simulink model "pmsm_model_dq"  (R2023b)
settings: Solver=VariableStepAuto  StartTime=0.0  StopTime=10.0  RelTol=1e-3
values from neighbouring files (symbols this model uses):
  B = 0.0000028    (= 2.8e-06)    [pm_params.m]
  J = 0.00016    [pm_params.m]
  Ld = 0.0057    [pm_params.m]
  Lq = 0.0125    [pm_params.m]
  pole = 4    [pm_params.m]
  Rs = 1.2    [pm_params.m]
undefined symbols (not defined in the file or in its folder): Lambda_f
settings Model: Creator=Yang  LastModifiedBy=Yang

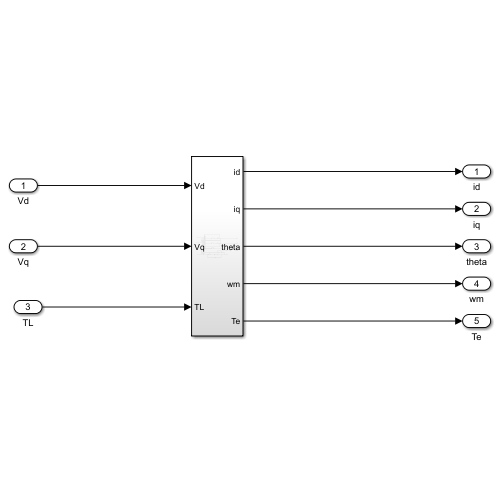
[thumbnail: Simulink's stored preview of the top-level diagram]
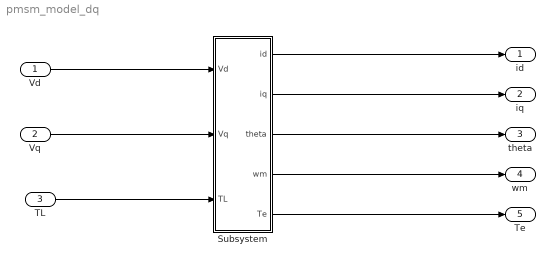
== system pmsm_model_dq ==
  Vd : Inport
  Vq : Inport  Port=2
  TL : Inport  Port=3
  Subsystem : Subsystem
  id : Outport
  iq : Outport  Port=2
  theta : Outport  Port=3
  wm : Outport  Port=4
  Te : Outport  Port=5
  wires:
  Vd/1 -> Subsystem/1(Vd)
  Vq/1 -> Subsystem/2(Vq)
  TL/1 -> Subsystem/3(TL)
  Subsystem/1(id) -> id/1
  Subsystem/2(iq) -> iq/1
  Subsystem/3(theta) -> theta/1
  Subsystem/4(wm) -> wm/1
  Subsystem/5(Te) -> Te/1

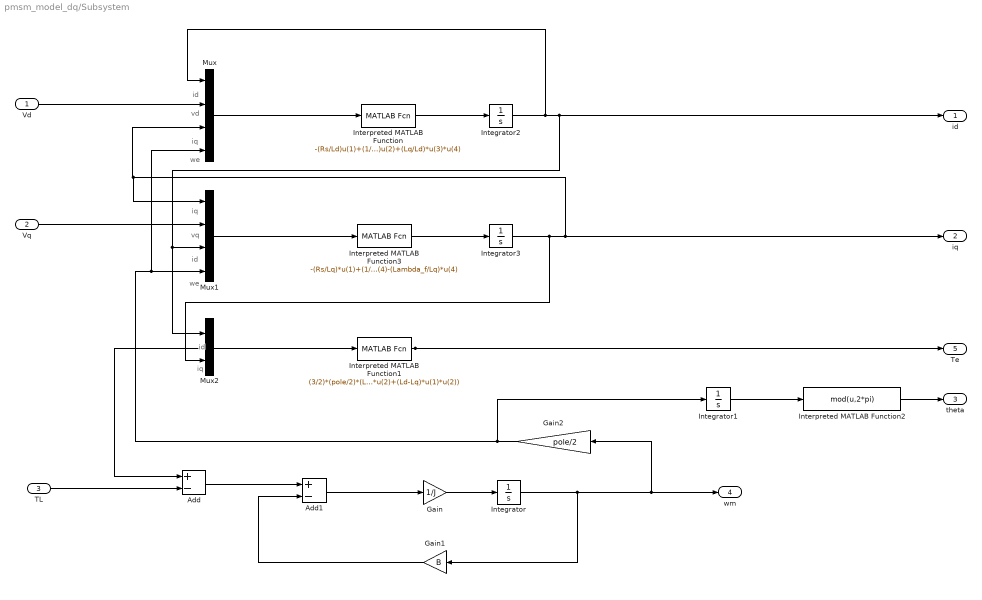
== system pmsm_model_dq/Subsystem ==
  note: iq
  note: id
  note: we
  note: id
  note: vq
  note: iq
  note: we
  note: iq
  note: vd
  note: id
  Vd : Inport
  Vq : Inport  Port=2
  TL : Inport  Port=3
  Add : Sum  Inputs=+-
  Add1 : Sum  Inputs=+-
  Gain : Gain  Gain=1/J
  Gain1 : Gain  Gain=B
  Gain2 : Gain  Gain=pole/2
  Integrator{,1..3} (4 alike) : Integrator
  Interpreted MATLAB Function : MATLABFcn  MATLABFcn=-(Rs/Ld)u(1)+(1/Ld)u(2)+(Lq/Ld)*u(3)*u(4)
  Interpreted MATLAB Function1 : MATLABFcn  MATLABFcn=(3/2)*(pole/2)*(Lambda_f*u(2)+(Ld-Lq)*u(1)*u(2))
  Interpreted MATLAB Function2 : MATLABFcn  MATLABFcn=mod(u,2*pi)
  Interpreted MATLAB Function3 : MATLABFcn  MATLABFcn=-(Rs/Lq)*u(1)+(1/Lq)u(2)-(Ld/Lq)*u(3)*u(4)-(Lambda_f/Lq)*u(4)
  Mux : Mux
  Mux1 : Mux
  Mux2 : Mux  Inputs=2
  id : Outport
  iq : Outport  Port=2
  theta : Outport  Port=3
  wm : Outport  Port=4
  Te : Outport  Port=5
  wires:
  Integrator1/1 -> Interpreted MATLAB Function2/1
  Integrator3/1 -> Mux2/2, iq/1, Mux1/1, Mux/3
  Interpreted MATLAB Function1/1 -> Te/1, Add/1
  Interpreted MATLAB Function/1 -> Integrator2/1
  Integrator/1 -> Gain1/1, wm/1, Gain2/1
  Interpreted MATLAB Function3/1 -> Integrator3/1
  Mux2/1 -> Interpreted MATLAB Function1/1
  Add/1 -> Add1/1
  Integrator2/1 -> Mux/1, id/1, Mux1/3, Mux2/1
  Gain2/1 -> Mux/4, Mux1/4, Integrator1/1
  Mux1/1 -> Interpreted MATLAB Function3/1
  Gain1/1 -> Add1/2
  Add1/1 -> Gain/1
  TL/1 -> Add/2
  Vd/1 -> Mux/2
  Gain/1 -> Integrator/1
  Mux/1 -> Interpreted MATLAB Function/1
  Interpreted MATLAB Function2/1 -> theta/1
  Vq/1 -> Mux1/2
